simulink model "dmass_sim_temp"  (R2023b)
settings: Solver=ode3  StartTime=0.0  StopTime=H  FixedStep=0.01  RelTol=1e-3
settings Model: Creator=jerome  LastModifiedBy=jerome
settings ModelReferenceCC: EnableRefExpFcnMdlSchedulingChecks=on

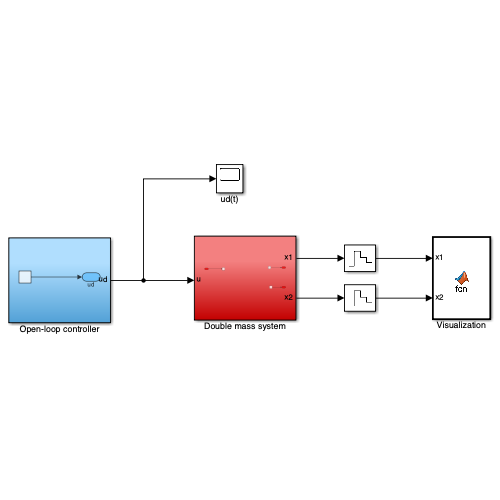
[thumbnail: Simulink's stored preview of the top-level diagram]
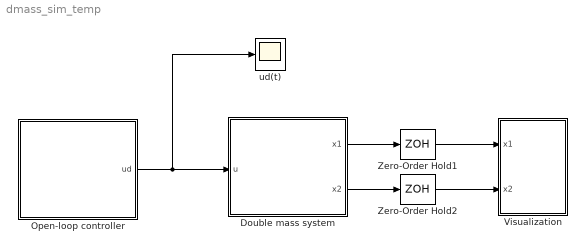
== system dmass_sim_temp ==
  Double mass system : Subsystem
  Open-loop controller : Subsystem
  Visualization : MATLAB Function  TreatAsAtomicUnit=on
  Zero-Order Hold1 : ZeroOrderHold  SampleTime=0.2
  Zero-Order Hold2 : ZeroOrderHold  SampleTime=0.2
  ud(t) : Scope
  wires:
  Open-loop controller/1(ud) -> ud(t)/1, Double mass system/1(u)
  Double mass system/1(x1) -> Zero-Order Hold1/1
  Zero-Order Hold2/1 -> Visualization/2(x2)
  Double mass system/2(x2) -> Zero-Order Hold2/1
  Zero-Order Hold1/1 -> Visualization/1(x1)

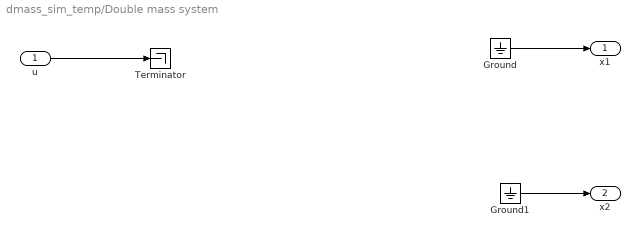
== system dmass_sim_temp/Double mass system ==
  u : Inport
  Ground : Ground
  Ground1 : Ground
  Terminator : Terminator
  x1 : Outport
  x2 : Outport  Port=2
  wires:
  u/1 -> Terminator/1
  Ground/1 -> x1/1
  Ground1/1 -> x2/1

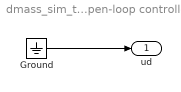
== system dmass_sim_temp/Open-loop controller ==
  Ground : Ground
  ud : Outport
  wires:
  Ground/1 -> ud/1

== matlab function dmass_sim_temp/Visualization ==
  data: x1 input; x2 input
function fcn(x1,x2)


so = 12; % spring offset
% mass 1
    Xmass1 = [ 5 ; 5 ; -5 ; -5 ; 5 ] + x1 - so;
    Ymass1 = [ -5 ; 5 ; 5 ; -5 ; -5]; 

% mass 2
    Xmass2 = [ 5 ; 5 ; -5 ; -5 ; 5 ] + x2 + so;
    Ymass2 = [ -5 ; 5 ; 5 ; -5 ; -5]; 

% the spring
    Xspring = [ 0 ; 4 ; 6 ; 10 ; 14 ; 18 ; 20 ; 24 ]/24*(x2-x1+2*so-10) + (x1-so+5);
    Yspring = [ 0 ; 0 ; 3 ; -3 ; 3 ; -3 ; 0 ; 0 ];

% to be able to use 'fill' even though the function is not supported for code generation
% see https://se.mathworks.com/help/simulink/slref/coder.extrinsic.html
coder.extrinsic('fill'); 

% draw the masses
fill(Xmass1,Ymass1,'r');
hold on
fill(Xmass2,Ymass2,'r');

% draw the spring
plot(Xspring,Yspring,'b','Linewidth',3);

% draw misc
plot([-so -so],[-10 -7],'k','Linewidth',2);  %draw a thin line at position x1 = 0
plot([so so],[-10 -7],'k','Linewidth',2);  %draw a thin line at position x2 = 0
hold off

axis([-20 60 -10 10]);
title('Mass-Spring-Damper system', 'FontSize',20);
axis equal;
grid on;

drawnow;
